simulink model "HOST_F103"  (R2020b)
settings: Solver=FixedStepDiscrete  StartTime=0.0  StopTime=inf  FixedStep=0.1  RelTol=1e-3
PreLoadFcn:
  | cd(fileparts(which(bdroot)));
InitFcn:
  | set_param([bdroot,'/refIq'], 'value','0');
  | set_param([bdroot,'/refRPM'], 'value', '0');
  | set_param([bdroot, '/cmd'], 'value', '0');
libraries: mcbhostblockslib x3
PreSaveFcn:
  | cd(fileparts(which(bdroot)));
settings Model: Creator=beau_  LastModifiedBy=beau_

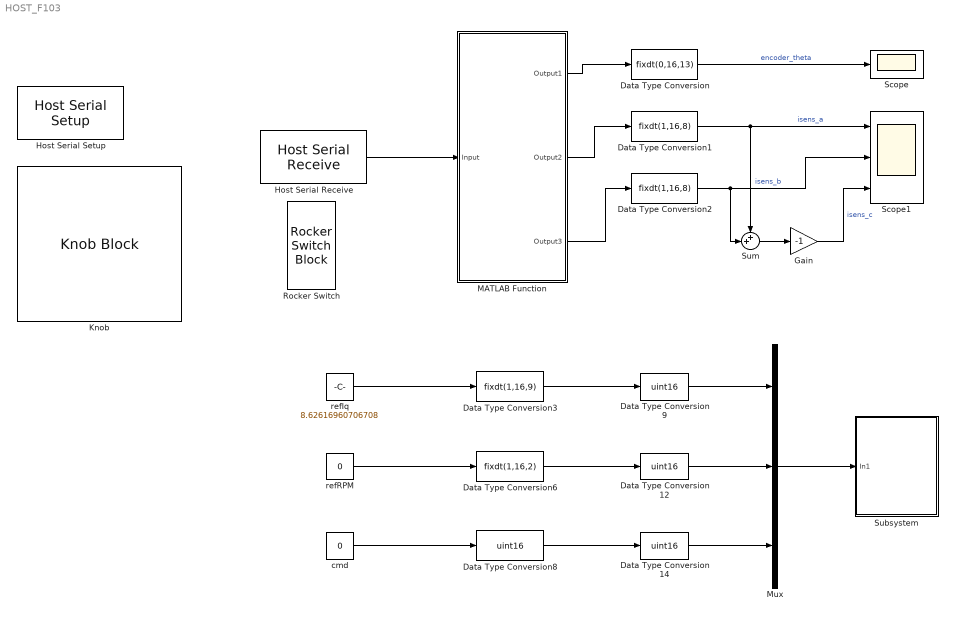
== system HOST_F103 ==
  Data Type Conversion : DataTypeConversion  OutDataTypeStr=fixdt(0,16,13)  ConvertRealWorld=Stored Integer (SI)
  Data Type Conversion1 : DataTypeConversion  OutDataTypeStr=fixdt(1,16,8)  ConvertRealWorld=Stored Integer (SI)
  Data Type Conversion12 : DataTypeConversion  OutDataTypeStr=uint16  ConvertRealWorld=Stored Integer (SI)
  Data Type Conversion14 : DataTypeConversion  OutDataTypeStr=uint16  ConvertRealWorld=Stored Integer (SI)
  Data Type Conversion2 : DataTypeConversion  OutDataTypeStr=fixdt(1,16,8)  ConvertRealWorld=Stored Integer (SI)
  Data Type Conversion3 : DataTypeConversion  OutDataTypeStr=fixdt(1,16,9)
  Data Type Conversion6 : DataTypeConversion  OutDataTypeStr=fixdt(1,16,2)
  Data Type Conversion8 : DataTypeConversion  OutDataTypeStr=uint16
  Data Type Conversion9 : DataTypeConversion  OutDataTypeStr=uint16  ConvertRealWorld=Stored Integer (SI)
  Gain : Gain  Gain=-1
  Host Serial Receive : mcbhostblockslib/Host Serial Receive  serialCon=Serial 1  dataHead='SS'  dataTail='EE'  dataType=int16  dataDim=[1000 3]  initValue=0  errOption=Output the last received value  errValue=0  sampleTime=0.1  outputStatus=off  blockingMode=on
      settings: SourceProductBaseCode=MT
  Host Serial Setup : mcbhostblockslib/Host Serial Setup  Priority=-99  comPortSer1='COM18'  baudRateA=2e6  charLenA=8  stopBitA=1  parityA=none  timeoutA=1.0  ByteOrderA=LittleEndian  comPortSer2='Please_select_a_port'  baudRateB=115200  charLenB=8  stopBitB=1  parityB=none  timeoutB=1.0  ByteOrderB=LittleEndian  comPortSer3='Please_select_a_port'  baudRateC=115200  charLenC=8  stopBitC=1  parityC=none  timeoutC=1.0  ByteOrderC=LittleEndian  comPortSer4='Please_select_a_port'  baudRateD=115200  charLenD=8  stopBitD=1  parityD=none  timeoutD=1.0  ByteOrderD=LittleEndian
      settings: SourceProductBaseCode=MT
  Knob : KnobBlock  ScaleMin=-10  ScaleMax=10
  MATLAB Function : MATLAB Function  TreatAsAtomicUnit=on
  Mux : Mux  Inputs=3
  Rocker Switch : RockerSwitchBlock
      settings: Values={{'Off', 'On'}, [0 1]}
  Scope : Scope
  Scope1 : Scope  NumInputPorts=3
  Subsystem : Subsystem  TreatAsAtomicUnit=on  SystemSampleTime=0.2
  Sum : Sum  Inputs=++|
  cmd : Constant  Value=0
  refIq : Constant  Value=8.62616960706708
  refRPM : Constant  Value=0
  wires:
  Host Serial Receive/1 -> MATLAB Function/1(Input)
  MATLAB Function/1(Output1) -> Data Type Conversion/1
  MATLAB Function/2(Output2) -> Data Type Conversion1/1
  MATLAB Function/3(Output3) -> Data Type Conversion2/1
  Mux/1 -> Subsystem/1(In1)
  Data Type Conversion/1 -> Scope/1  "encoder_theta"
  Data Type Conversion1/1 -> Scope1/1, Sum/1  "isens_a"
  Data Type Conversion2/1 -> Sum/2, Scope1/2  "isens_b"
  refIq/1 -> Data Type Conversion3/1
  refRPM/1 -> Data Type Conversion6/1
  cmd/1 -> Data Type Conversion8/1
  Data Type Conversion8/1 -> Data Type Conversion14/1
  Data Type Conversion14/1 -> Mux/3
  Data Type Conversion3/1 -> Data Type Conversion9/1
  Data Type Conversion9/1 -> Mux/1
  Data Type Conversion6/1 -> Data Type Conversion12/1
  Data Type Conversion12/1 -> Mux/2
  Sum/1 -> Gain/1
  Gain/1 -> Scope1/3  "isens_c"

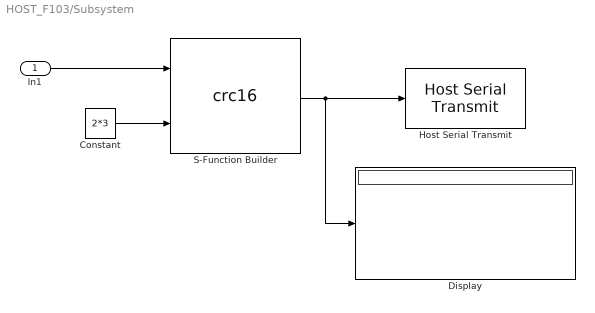
== system HOST_F103/Subsystem ==
  In1 : Inport
  Constant : Constant  Value=2*3  OutDataTypeStr=single  SampleTime=-1
  Display : Display
  Host Serial Transmit : mcbhostblockslib/Host Serial Transmit  serialCon=Serial 1  header=''  tail=''  enableBlockingMode=off
      settings: SourceProductBaseCode=MT
  S-Function Builder : S-Function  FunctionName=crc16  SFunctionModules=crc16_wrapper  SFunctionDeploymentMode=off  EnableBusSupport=off  mask(S-Function Builder){}
      mask help: Simulink:masks:SFunctionBuilder_MD
      mask init:
      | val = [[.9  0.75 0.75 1 1 .9 .9 1]',[1 1 0.75 0.75 .9 .9 1 .9]'];try , sys = get_param(gcb,'SfunBuilderFcnName');if isempty(sys), sys = get_param(gcb,'FunctionName'); end,catch, sys = get_param(gcb,'FunctionName'); end
      settings: CopyFcn=set_param(gcbh,'LinkStatus','none')  OpenFcn=sfunctionwizard(gcbh)
      mask Display: plot(val(:,1),val(:,2)),disp(sys),port_label('input',1,'ptr'),port_label('input',2,'bytes'),port_label('output',1,'crcOut')
  wires:
  Constant/1 -> S-Function Builder/2
  S-Function Builder/1 -> Display/1, Host Serial Transmit/1
  In1/1 -> S-Function Builder/1

== matlab function HOST_F103/MATLAB Function ==
  data: Input input; Output1 output; Output2 output; Output3 output
function [Output1,Output2,Output3]  = unBuf(Input)

Output1 = Input(:, 1);
Output2 = Input(:, 2);
Output3 = Input(:, 3);
end
